simulink model "ZiemskiAlgorytmRozszerzony"  (R2017a)
settings: Solver=ode113  StartTime=0.0  StopTime=10.0  RelTol=1e-2
values from neighbouring files (symbols this model uses):
  param = evalin('base','param')    [getSaveInfo.m]    (also in loadBackUp.m)
(part 1 of 3)
settings Model: Creator=www  LastModifiedBy=www
settings SolverCC: MaxConsecutiveMinStep=1000  ShapePreserveControl=EnableAll  ZeroCrossAlgorithm=Adaptive
settings DataIOCC: SaveOutput=off  SignalLogging=off  DSMLogging=off  SaveTime=off

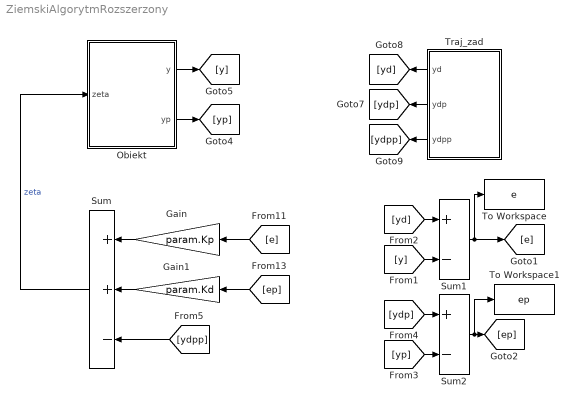
== system ZiemskiAlgorytmRozszerzony ==
  Gain : Gain  Gain=param.Kp
  Gain1 : Gain  Gain=param.Kd
  Obiekt : Subsystem
  Sum : Sum  Inputs=++-
  Sum1 : Sum  Inputs=+-
  Sum2 : Sum  Inputs=+-
  To Workspace : ToWorkspace  VariableName=e  SaveFormat=Timeseries  SampleTime=-1
  To Workspace1 : ToWorkspace  VariableName=ep  SaveFormat=Timeseries  SampleTime=-1
  Traj_zad : Subsystem
  wires:
  Gain/1 -> Sum/1
  Gain1/1 -> Sum/2
  [e] -> Gain/1
  Obiekt/2(yp) -> [yp]
  Obiekt/1(y) -> [y]
  [ep] -> Gain1/1
  Sum2/1 -> To Workspace1/1, [ep]
  Sum1/1 -> To Workspace/1, [e]
  [ydp] -> Sum2/1
  [yp] -> Sum2/2
  [y] -> Sum1/2
  [yd] -> Sum1/1
  [ydpp] -> Sum/3
  Traj_zad/1(yd) -> [yd]
  Traj_zad/3("ydpp ") -> [ydpp]
  Traj_zad/2(ydp) -> [ydp]
  Sum/1 -> Obiekt/1(zeta)  "zeta"

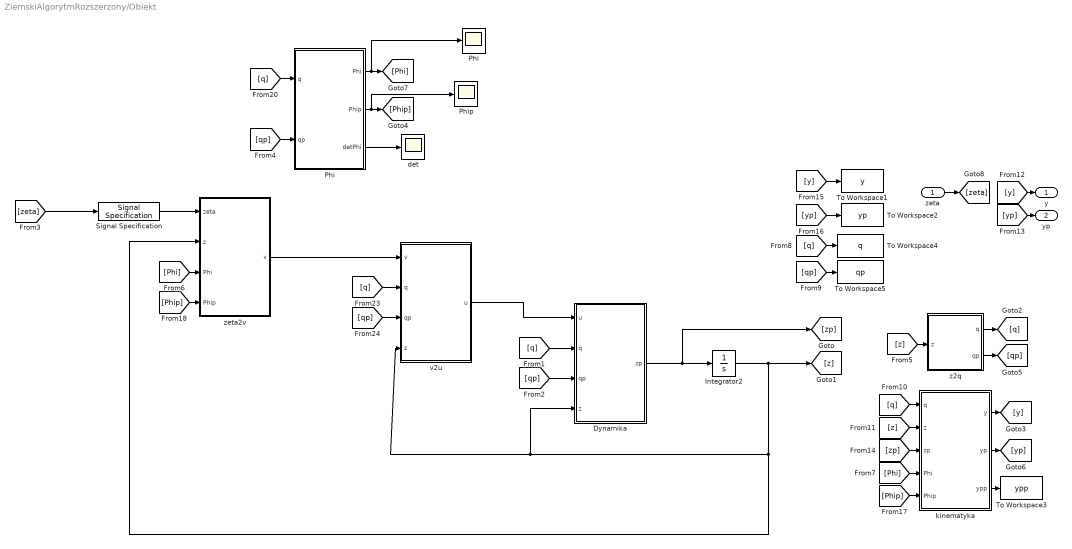
== system ZiemskiAlgorytmRozszerzony/Obiekt ==
  zeta : Inport
  Dynamika : MATLAB Function  TreatAsAtomicUnit=on
  Integrator2 : Integrator  InitialCondition=param.initCond.z0
  Phi : MATLAB Function  TreatAsAtomicUnit=on
  "Phi   " : Scope
  Phip : Scope
  Signal Specification : SignalSpecification  Dimensions=[5 1]
  To Workspace1 : ToWorkspace  VariableName=y  SaveFormat=Timeseries  SampleTime=-1
  To Workspace2 : ToWorkspace  VariableName=yp  SaveFormat=Timeseries  SampleTime=-1
  To Workspace3 : ToWorkspace  VariableName=ypp  SaveFormat=Timeseries  SampleTime=-1
  To Workspace4 : ToWorkspace  VariableName=q  SaveFormat=Timeseries  SampleTime=-1
  To Workspace5 : ToWorkspace  VariableName=qp  SaveFormat=Timeseries  SampleTime=-1
  det : Scope
  kinematyka : MATLAB Function  TreatAsAtomicUnit=on
  v2u : MATLAB Function  TreatAsAtomicUnit=on
  z2q : Subsystem
  zeta2v : MATLAB Function  TreatAsAtomicUnit=on
  y : Outport
  yp : Outport  Port=2
  wires:
  [q] -> Dynamika/2(q)
  Dynamika/1(zp) -> Integrator2/1, [zp]
  [z] -> z2q/1(z)
  [zeta] -> Signal Specification/1
  [qp] -> v2u/3(qp)
  zeta/1 -> [zeta]
  Integrator2/1 -> zeta2v/2(z), v2u/4(z), Dynamika/4(z), [z]
  [qp] -> Dynamika/3(qp)
  [Phip] -> zeta2v/4(Phip)
  zeta2v/1(v) -> v2u/1(v)
  v2u/1(u) -> Dynamika/1(u)
  Signal Specification/1 -> zeta2v/1(zeta)
  [q] -> v2u/2(q)
  z2q/1(q) -> [q]
  [zp] -> kinematyka/3(zp)
  [z] -> kinematyka/2(z)
  [q] -> To Workspace4/1
  z2q/2(qp) -> [qp]
  [yp] -> yp/1
  [yp] -> To Workspace2/1
  [y] -> To Workspace1/1
  kinematyka/1(y) -> [y]
  kinematyka/3(ypp) -> To Workspace3/1
  [y] -> y/1
  [qp] -> To Workspace5/1
  kinematyka/2(yp) -> [yp]
  [q] -> kinematyka/1(q)
  [q] -> Phi/1(q)
  [qp] -> Phi/2(qp)
  [Phi] -> zeta2v/3(Phi)
  [Phi] -> kinematyka/4(Phi)
  [Phip] -> kinematyka/5(Phip)
  Phi/2(Phip) -> Phip/1, [Phip]
  Phi/1(Phi) -> "Phi   "/1, [Phi]
  Phi/3(detPhi) -> det/1

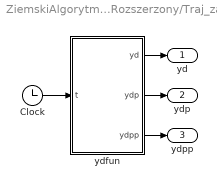
== system ZiemskiAlgorytmRozszerzony/Traj_zad ==
  Clock : Clock
  ydfun : MATLAB Function  TreatAsAtomicUnit=on
  yd : Outport
  ydp : Outport  Port=2
  "ydpp " : Outport  Port=3
  wires:
  ydfun/2(ydp) -> ydp/1
  ydfun/3(ydpp) -> "ydpp "/1
  ydfun/1(yd) -> yd/1
  Clock/1 -> ydfun/1(t)

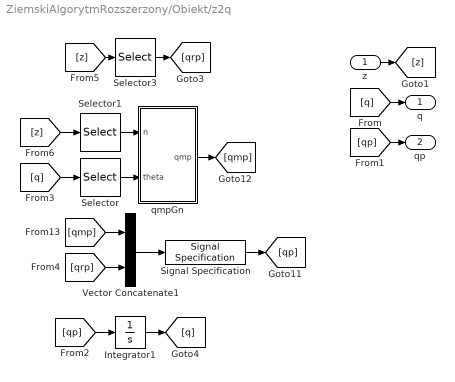
== system ZiemskiAlgorytmRozszerzony/Obiekt/z2q ==
  z : Inport
  Integrator1 : Integrator  InitialCondition=[param.initCond.q0]
  Selector : Selector  InputPortWidth=8  IndexOptions=Index vector (dialog)  Indices=[3]  OutputSizes=1
  Selector1 : Selector  InputPortWidth=5  IndexOptions=Index vector (dialog)  Indices=[1 2]  OutputSizes=1
  Selector3 : Selector  InputPortWidth=5  IndexOptions=Index vector (dialog)  Indices=[3 4 5]  OutputSizes=1
  Signal Specification : SignalSpecification  Dimensions=[8 1]
  Vector Concatenate1 : Concatenate
  qmpGn : MATLAB Function  TreatAsAtomicUnit=on
  q : Outport
  qp : Outport  Port=2
  wires:
  z/1 -> [z]
  [q] -> q/1
  [qp] -> qp/1
  [z] -> Selector1/1
  Selector/1 -> qmpGn/2(theta)
  Selector3/1 -> [qrp]
  [z] -> Selector3/1
  [qp] -> Integrator1/1
  Integrator1/1 -> [q]
  [q] -> Selector/1
  Selector1/1 -> qmpGn/1(n)
  qmpGn/1(qmp) -> [qmp]
  [qmp] -> Vector Concatenate1/1
  [qrp] -> Vector Concatenate1/2
  Vector Concatenate1/1 -> Signal Specification/1
  Signal Specification/1 -> [qp]

== matlab function ZiemskiAlgorytmRozszerzony/Obiekt/z2q/qmpGn ==
  data: n input; qmp output; theta input
function qmp = fcn(n,theta)
L=0.3;
R=0.075;
qmp=[cos(theta), cos(theta);
    sin(theta), sin(theta)
    1/L, -1/L;
    2/R, 0;
    0, 2/R]*n;
